simulink model "ECU_Trunk_Lid_Logic_Model"  (R2024a)
settings: Solver=VariableStepAuto  StartTime=0.0  StopTime=10.0  RelTol=1e-3
settings Model: Creator=ec97883  LastModifiedBy=ec97883

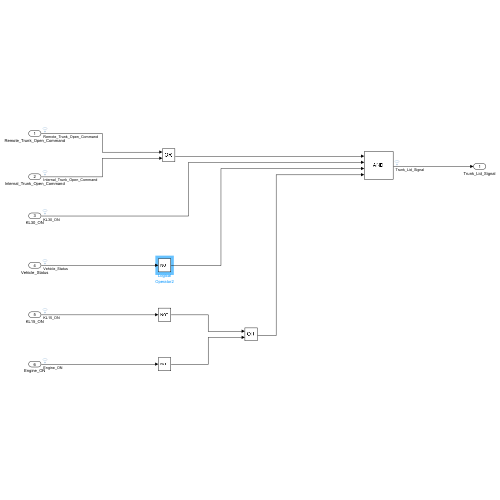
[thumbnail: Simulink's stored preview of the top-level diagram]
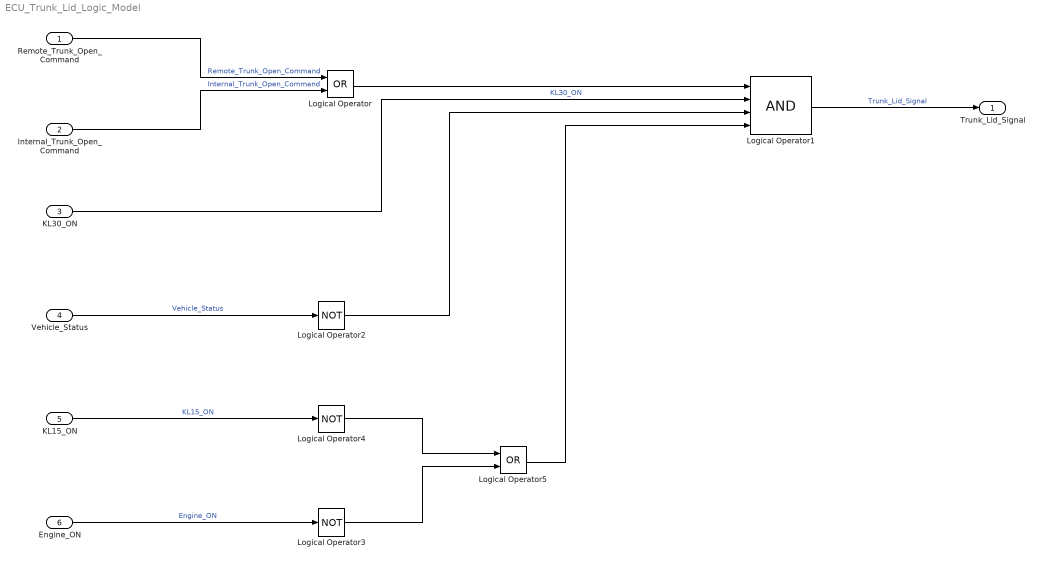
== system ECU_Trunk_Lid_Logic_Model ==
  Remote_Trunk_Open_Command : Inport  OutDataTypeStr=boolean  PortDimensions=1
  Internal_Trunk_Open_Command : Inport  Port=2  OutDataTypeStr=boolean  PortDimensions=1
  KL30_ON : Inport  Port=3  OutDataTypeStr=boolean  PortDimensions=1
  Vehicle_Status : Inport  Port=4  OutDataTypeStr=boolean  PortDimensions=1
  KL15_ON : Inport  Port=5  OutDataTypeStr=boolean  PortDimensions=1
  Engine_ON : Inport  Port=6  OutDataTypeStr=boolean  PortDimensions=1
  Logical Operator : Logic  Operator=OR  AllPortsSameDT=off  OutDataTypeStr=boolean
  Logical Operator1 : Logic  Inputs=4  AllPortsSameDT=off  OutDataTypeStr=boolean
  Logical Operator2 : Logic  Operator=NOT  AllPortsSameDT=off  OutDataTypeStr=boolean
  Logical Operator3 : Logic  Operator=NOT  AllPortsSameDT=off  OutDataTypeStr=boolean
  Logical Operator4 : Logic  Operator=NOT  AllPortsSameDT=off  OutDataTypeStr=boolean
  Logical Operator5 : Logic  Operator=OR  AllPortsSameDT=off  OutDataTypeStr=boolean
  Trunk_Lid_Signal : Outport  OutDataTypeStr=boolean  PortDimensions=1
  wires:
  Remote_Trunk_Open_Command/1 -> Logical Operator/1  "Remote_Trunk_Open_Command"
  Internal_Trunk_Open_Command/1 -> Logical Operator/2  "Internal_Trunk_Open_Command"
  Logical Operator/1 -> Logical Operator1/1
  KL30_ON/1 -> Logical Operator1/2  "KL30_ON"
  Vehicle_Status/1 -> Logical Operator2/1  "Vehicle_Status"
  KL15_ON/1 -> Logical Operator4/1  "KL15_ON"
  Engine_ON/1 -> Logical Operator3/1  "Engine_ON"
  Logical Operator4/1 -> Logical Operator5/1
  Logical Operator3/1 -> Logical Operator5/2
  Logical Operator5/1 -> Logical Operator1/4
  Logical Operator1/1 -> Trunk_Lid_Signal/1  "Trunk_Lid_Signal"
  Logical Operator2/1 -> Logical Operator1/3
